simulink library "pmm"  (R2021b)
settings: Solver=VariableStepAuto  StartTime=0.0  StopTime=10.0  RelTol=1e-3
undefined symbols (not defined in the file or in its folder): APMM_CoolgFanActCurr_X_pct, APMM_EWP1Curr_X_c, APMM_EWP3Curr_X_c, APMM_LVBattChktime_X_enum, APMM_LVBattChrgtime_X_enum, APMM_LVChrgLv24V_X_mV, APMM_LVChrgLv_X_mV, ENUM_ANTITHEFT_ALARM, ENUM_ANTITHEFT_ARM, ENUM_ANTITHEFT_DISARM, ENUM_ANTITHEFT_WAIT, ENUM_CHRGPLUGSTA_NONE, ENUM_CRASHSTATE_NOCRASH, ENUM_DCDCFAULTSTA_ANYFAULTLV1, ENUM_DCDCFAULTSTA_ANYFAULTLV2, ENUM_DRIVETRAIN_AWD, ENUM_DRIVETRAIN_FWD, ENUM_DRIVETRAIN_RWD, ENUM_EBSBRKSW_PRESSED, ENUM_GEARACTUALPOSN_D, ENUM_GEARACTUALPOSN_N, ENUM_GEARACTUALPOSN_P, ENUM_GEARACTUALPOSN_R, ENUM_HVBATTREADYPRE_READY, ENUM_PDKEYRAWLULOCK_INLOCK, ENUM_PDKEYRAWLULOCK_INUNLOCK, ENUM_PDKEYRAWPS_INPS, ENUM_PDKEYSTA_LOCK, ENUM_PDKEYSTA_PS, ENUM_PDKEYSTA_UNAVALIABLE, ENUM_PDKEYSTA_UNLOCK, ENUM_POWERSTA_OFF, ENUM_POWERSTA_OFFA, ENUM_POWERSTA_OFFC, ENUM_POWERSTA_ON, ENUM_POWERSTA_READY, ENUM_POWERSTA_STANDBY, ENUM_PWRSTASW_PWRUP, ENUM_PWRSTASW_READY, FALSE, KPMM_AllDoorClosedHoldTime_s, KPMM_APSAllowThd_pct, KPMM_BattDownFailtime_s, KPMM_BattUpFailtime_s, KPMM_BattUpResetRty_cnt, KPMM_BattUpResetSW_flg, KPMM_BattUpResetTO_s, KPMM_BattUpRstDlyTO_s, KPMM_BrakeSWHoldTime_s, KPMM_ChrgPlugHoldTime_s, KPMM_DCDCDisableFailtime_s, KPMM_DCDCEnableFailtime_s, KPMM_DCDCVSET_V, KPMM_DCDCVSETLVChrg_V, KPMM_DoorSWHoldTime_s, KPMM_DriverSafetyChkFailtime_s, KPMM_DrivetrainSelect_enum_ovrdflg, KPMM_DrivetrainSelect_enum_ovrdval, KPMM_FDADC12VDetAccu_s, KPMM_FDADC12VDetAccuIntval_s ... (+60)
libraries: simulink x35, hcu_lib x13
(part 2 of 6)

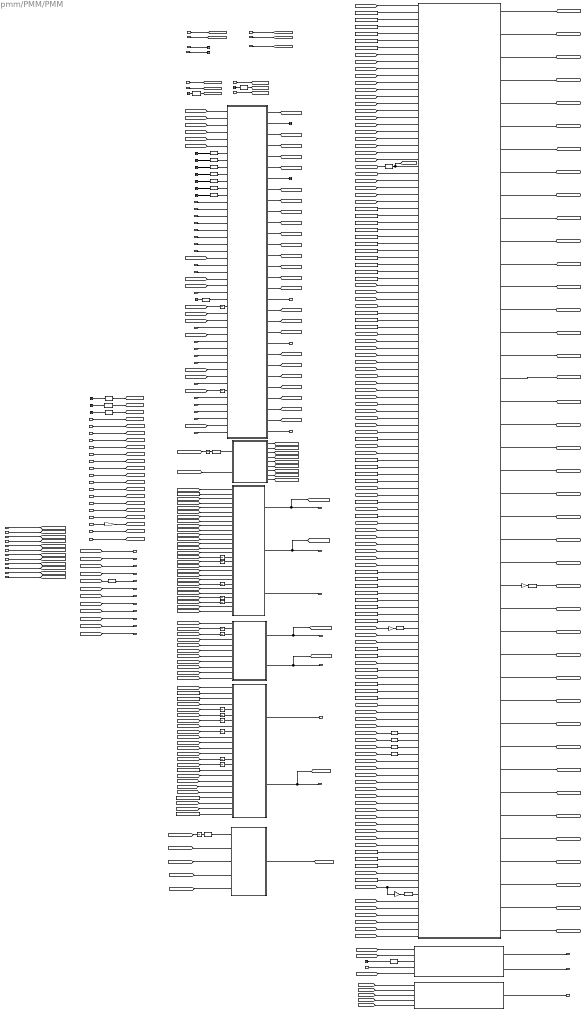
== system pmm/PMM/PMM ==
  note: BMS
  note: PEU
  note: 0 = open; 1 = close
  task_time_s : Inport
  VINP_SeatSW_flg : Inport  Port=2
  VINP_HoodSW_flg : Inport  Port=3
  VINP_TailgateSW_flg : Inport  Port=4
  VINP_PBSWGPIO_flg : Inport  Port=5
  VINP_IVIPwroffreq_flg : Inport  Port=6
  VINP_IVITriggerreq_flg : Inport  Port=7
  VINP_OFFACMODE_enum : Inport  Port=8
  VINP_AVMOFFRecButt_flg : Inport  Port=9
  VINP_SchedChgwake_flg : Inport  Port=10
  VINP_SchedChgbutt_flg : Inport  Port=11
  VINP_PWCONTINUEUSE_flg : Inport  Port=12
  VINP_DCDCReady4Pre_flg : Inport  Port=13
  VINP_DCDCEnabled_flg : Inport  Port=14
  VINP_OBCEnabled_flg : Inport  Port=15
  VINP_OBCReady4Pre_flg : Inport  Port=16
  VINP_OBCFaultStatus_enum : Inport  Port=17
  VINP_DCDCAuxVolt_V : Inport  Port=18
  VINP_RrMCUDCBusVolt_V : Inport  Port=19
  VINP_RrMCUDischrgSta_flg : Inport  Port=20
  VINP_RrMCUEnaSta_flg : Inport  Port=21
  VINP_RrMCUErr_enum : Inport  Port=22
  VINP_RrMCUReady4Pre_flg : Inport  Port=23
  VINP_RrMCUReady_flg : Inport  Port=24
  VINP_RrMCUTemp_C : Inport  Port=25
  VINP_HVBattReady4Pre_enum : Inport  Port=26
  VINP_ChrgPlugSta_enum : Inport  Port=27
  VINP_BMSREADY_flg : Inport  Port=28
  VINP_HVILSta_flg : Inport  Port=29
  VINP_HVBContactorSta_flg : Inport  Port=30
  VINP_ExtChrgSta_enum : Inport  Port=31
  VINP_HVBattSOC_pct : Inport  Port=32
  VINP_RrTMSpd_rpm : Inport  Port=33
  VINP_OBCPluginSta_flg : Inport  Port=34
  VINP_BMSWarn5_flg : Inport  Port=35
  VINP_BMSWarn6_flg : Inport  Port=36
  VINP_BMSWarn7_flg : Inport  Port=37
  VINP_BMSWarn8_flg : Inport  Port=38
  VINP_HVBPreheatPrecoolSta_enum : Inport  Port=39
  VINP_DCDCFaultSta_enum : Inport  Port=40
  VINP_CANMsgValidBMS5_flg : Inport  Port=41
  VINP_CANMsgValidBMS3_flg : Inport  Port=42
  VINP_RrEDURealTMTq_Nm : Inport  Port=43
  VINP_DCDCAuxCur_A : Inport  Port=44
  VINP_V2LSta_enum : Inport  Port=45
  VINP_LVBattDet12V_V : Inport  Port=46
  VINP_PDKeyAreaPS_flg : Inport  Port=47
  VINP_PDKeyAreaLockUnlock_flg : Inport  Port=48
  VINP_CANMsgValidDKC1_flg : Inport  Port=49
  VINP_PowerOffTSet_cnt : Inport  Port=50
  VINP_RePwrReqTbox_enum : Inport  Port=51
  VTQD_GearActualPosn_enum : Inport  Port=52
  VTQD_PBWLockTO_flg : Inport  Port=53
  VBCM_AntitheftSta_enum : Inport  Port=54
  VINP_AllowMovThd_OTA_enum : Inport  Port=55
  VINP_PwrReq_OTA_enum : Inport  Port=56
  VINP_DrivetrainSelect_enum : Inport  Port=57
  VINP_EvccAplusPwrUpReq_flg : Inport  Port=58
  VDHP_ActAPSPosn_pct : Inport  Port=59
  VDHP_EAPS12RangeSta_enum : Inport  Port=60
  VINP_FDEWP1Cmd_enum : Inport  Port=61
  VINP_FDEWP3Cmd_enum : Inport  Port=62
  VINP_CoolgFanActDuty_pct : Inport  Port=63
  VINP_PowerOffTSetDKC_enum : Inport  Port=64
  VINP_RePwrReqDKCT_enum : Inport  Port=65
  VDKC_KeyAreaLockUnlock_enum : Inport  Port=66
  VDKC_KeyAreaPS_enum : Inport  Port=67
  VINP_FASpeed_kph : Inport  Port=68
  VINP_PDUDCDCRlySta_enum : Inport  Port=69
  VINP_PDUEACRlySta_enum : Inport  Port=70
  VINP_PDUEHPSRlySta_enum : Inport  Port=71
  VINP_DCDCEnSta_enum : Inport  Port=72
  VINP_EACEnSta_enum : Inport  Port=73
  VINP_EHPSEnSta_enum : Inport  Port=74
  VINP_EBSBrakeSW_enum : Inport  Port=75
  VINP_PDUSelfChkSta_flg : Inport  Port=76
  VINP_LVBattDet24V_V : Inport  Port=77
  VINP_CANMsgValidDCDCStatus2_flg : Inport  Port=78
  VINP_FDDoorOpen_enum : Inport  Port=79
  VACC_EACPreSelfChkSta_flg : Inport  Port=80
  BoringSpec : Subsystem
  Cast To Boolean : DataTypeConversion  OutDataTypeStr=boolean
  Cast To Boolean1 : DataTypeConversion  OutDataTypeStr=boolean
  Cast To Boolean2 : DataTypeConversion  OutDataTypeStr=boolean
  Constant : Constant  Value=KPMM_LVBattChkOKStdT_s
  Constant1 : Constant  Value=KPMM_LVBattThd_V
  Constant10 : Constant  Value=KPMM_OBCDisableFailtime_s
  Constant11 : Constant  Value=KPMM_DriverSafetyChkFailtime_s
  Constant12 : Constant  Value=KPMM_FDADC12VDetAccu_s
  Constant13 : Constant  Value=KPMM_PrechrgChkFailtime_s
  Constant14 : Constant  Value=KPMM_FirstLVCheckHoldT_s
  Constant15 : Constant  Value=KPMM_MLvSafetyFailtime_s
  Constant16 : Constant  Value=KPMM_MCUDisChrgFailtime_s
  Constant17 : Constant  Value=KPMM_DCDCVSET_V
  Constant18 : Constant  Value=KPMM_OFFStaByPassLVBatt_flg
  Constant19 : Constant  Value=KPMM_SilentChrgReq_flg_ovrdflg
  Constant2 : Constant  Value=KPMM_PwrStaStdTO_s
  Constant20 : Constant  Value=KPMM_DCDCEnableFailtime_s
  Constant21 : Constant  Value=KPMM_BattDownFailtime_s
  Constant22 : Constant  Value=KPMM_MCUDisableFailtime_s
  Constant23 : Constant  Value=KPMM_APSAllowThd_pct
  Constant24 : Constant  Value=KPMM_DCDCDisableFailtime_s
  Constant25 : Constant  Value=KPMM_SilentChrgReq_flg_ovrdval
  Constant26 : Constant  Value=KPMM_HVBattSOCThd_pct
  Constant27 : Constant  Value=KPMM_HVSOCWarnThd_pct
  Constant28 : Constant  Value=KPMM_HVBattSOCPwrDwnThd_pct
  Constant29 : Constant  Value=KPMM_HVSOCWarnThd_pct
  Constant3 : Constant  Value=KPMM_HVBattSOCThd_pct
  Constant30 : Constant  Value=KPMM_OffA2OffTime_s
  Constant31 : Constant  Value=KPMM_PluginVehSpdThd_kph
  Constant32 : Constant  Value=KPMM_LVChrgCurrMthd_flg
  Constant33 : Constant  Value=KPMM_LVChrgHoldT_s
  Constant34 : Constant  Value=KPMM_SysBaseCurr_A
  Constant35 : Constant  Value=KPMM_HVSOCWarnTime_s
  Constant36 : Constant  Value=KPMM_SilentChrgReqTO_s
  Constant37 : Constant  Value=KPMM_PwrStaONTOPop_s
  Constant38 : Constant  Value=KPMM_LVBattChkWakehold_s
  Constant39 : Constant  Value=KPMM_LVBattOFFSlpThd_mV
  Constant4 : Constant  Value=KPMM_HVBSOCOffStaChkFailtime_s
  Constant40 : Constant  Value=KPMM_OFFLVBattChkRetry_cnt
  Constant41 : Constant  Value=KPMM_SysPwrDownDbns_s
  Constant42 : Constant  Value=KPMM_BattUpResetRty_cnt
  Constant43 : Constant  Value=KPMM_BattUpResetSW_flg
  Constant44 : Constant  Value=KPMM_BattUpResetTO_s
  Constant45 : Constant  Value=KPMM_BattUpRstDlyTO_s
  Constant46 : Constant  Value=KPMM_HoodOffChkFailtime_s
  Constant47 : Constant  Value=KPMM_FDADC24VDetAccu_s
  Constant48 : Constant  Value=KPMM_FDADC24VDetAccuIntval_s
  Constant49 : Constant  Value=KPMM_LVBattOFFSlpThd24V_mV
  Constant5 : Constant  Value=KPMM_HVBSOCOFFCStaChkFailtime_s
  Constant50 : Constant  Value=KPMM_LVBattThd24V_V
  Constant6 : Constant  Value=KPMM_FDADC12VDetAccuIntval_s
  Constant7 : Constant  Value=KPMM_OBCPreChgChkFailtime_s
  Constant8 : Constant  Value=KPMM_SafetyChkFailtime_s
  Constant9 : Constant  Value=KPMM_BattUpFailtime_s  OutDataTypeStr=single
  DCDC output volt setpoint judgment : Subsystem
  Data Type Conversion : DataTypeConversion
  Data Type Conversion1 : DataTypeConversion
  Data Type Conversion{3,5,10,15} (4 alike) : DataTypeConversion  OutDataTypeStr=uint8
  Data Type Conversion{7..9,11..12} (5 alike) : DataTypeConversion  OutDataTypeStr=boolean
  Data Type Conversion{2,4,6,13..14,16} (6 alike) : DataTypeConversion  OutDataTypeStr=single
  Data Type Conversion39 : DataTypeConversion
  Detect Decrease : simulink/Logic and Bit Operations/Detect Decrease  vinit=0.0  OutDataTypeStr=boolean
  Detect Increase : simulink/Logic and Bit Operations/Detect Increase  vinit=0.0  OutDataTypeStr=boolean
  Detect Increase1 : simulink/Logic and Bit Operations/Detect Increase  vinit=0.0  OutDataTypeStr=boolean
  Detect Increase2 : simulink/Logic and Bit Operations/Detect Increase  vinit=0.0  OutDataTypeStr=boolean
  Gain : Gain  Gain=MIN2SEC
  Gain1 : Gain  Gain=1000
  Gain2 : Gain  Gain=0.001
  Gain3 : Gain  Gain=1000
  Ground{,1..13} (14 alike) : Ground
  MCU_EnaReq_Control : Subsystem
  PMMDataConvert : Subsystem  AncestorBlock=pmm/PMM/PowerModeManagement/PMMDataConvert
  PMM_State_Machine : Stateflow chart  TreatAsAtomicUnit=on
      settings: PortSchema="{\"entries\":[{\"content\":{\"sides\":[{\"content\":{\"connectorIds\":[\"In1\",\"In2\",\"In3\",\"In4\",\"In5\",\"In6\",\"In7\",\"In8\",\"In9\",\"In10\",\"In11\",\"In12\",\"In13\",\"In14\",\"In15\",\"In16\",\"In17\",\"In18\",\"In19\",\"In20\",\"In21\",\"In22\",\"In23\",\"In24\",\"In25\",\"In26\",\"In27\",\"In28\",\"In29\",\"In30\",\"In31\",\"In32\",\"In33\",\"In34\",\"In35\",\"In36\",\"In37\",\"In38\",\"In39\",\"In40\",\"In41\",\"In42\",\"In43\",\"In44\",\"In45\",\"In46\",\"In47\",\"In48\",\"In49\",\"In50\",\"In52\",\"In53\",\"In54\",\"In55\",\"In56\",\"In57\",\"In58\",\"In51\",\"In59\",\"In60\",\"In61\",\"In62\",\"In63\",\"In65\",\"In66\",\"In67\",\"In68\",\"In69\",\"In70\",\"In73\",\"In74\",\"In71\",\"In72\",\"In64\",\"In75\",\"In76\",\"In77\",\"In78\",\"In79\",\"In80\",\"In81\",\"In82\",\"In83\",\"In84\",\"In85\",\"In86\",\"In87\",\"In88\",\"In89\",\"In90\",\"In96\",\"In97\",\"In98\",\"In99\",\"In100\",\"In95\",\"In91\",\"In92\",\"In93\",\"In94\",\"In101\",\"In102\",\"In103\",\"In104\",\"In105\",\"In106\",\"In107\",\"In108\",\"In109\",\"In110\",\"In111\",\"In112\",\"In113\",\"In114\",\"In115\",\"In116\",\"In117\",\"In118\",\"In119\",\"In120\",\"In121\",\"In123\",\"In124\",\"In125\",\"In126\",\"In127\",\"In128\",\"In122\",\"In129\",\"In130\",\"In131\",\"In132\",\"In133\",\"In134\"]},\"type\":\"ConnectorPlacement.EquallySpacedRectSide\",\"uuid\":\"8ab1b0ff-73ed-4b41-8f3f-fcf16c31188d\"},{\"content\":{\"connectorIds\":[\"Out1\",\"Out2\",\"Out3\",\"Out4\",\"Out5\",\"Out6\",\"Out7\",\"Out8\",\"Out9\",\"Out10\",\"Out11\",\"Out12\",\"Out13\",\"Out14\",\"Out17\",\"Out18\",\"Out19\",\"Out20\",\"Out21\",\"Out22\",\"Out23\",\"Out24\",\"Out25\",\"Out26\",\"Out27\",\"Out28\",\"Out29\",\"Out30\",\"Out31\",\"Out32\",\"Out33\",\"Out34\",\"Out35\",\"Out15\",\"Out16\",\"Out36\",\"Out37\",\"Out38\",\"Out40\",\"Out41\",\"Out39\"],\"side\":\"RIGHT\"},\"type\":\"ConnectorPlacement.EquallySpacedRectSide\",\"uuid\":\"e75ad163-33ee-46d6-b33a-670f57cb3f5e\"},{\"content\":{\"connectorIds\":[],\"side\":\"TOP\"},\"type\":\"ConnectorPlacement.EquallySpacedRectSide\",\"uuid\":\"84c68278-d5af-48d1-859e-0f05090acbaa\"}]},\"type\":\"ConnectorPlacement.EquallySpacedConnector\",\"uuid\":\"278d3476-0e07-485b-a357-39a0667eafe4\"}],\"packageUris\":[\"http://schema.mathworks.com/mf0/Connector/R2020b\"],\"version\":\"1.0\"}"
  PushButton_Handle : Subsystem
  RequirementManagementForPowerDown : Stateflow chart  TreatAsAtomicUnit=on
  RequirementManagementForPowerStateConstrain : Stateflow chart  TreatAsAtomicUnit=on
      settings: PortSchema="{\"entries\":[{\"content\":{\"sides\":[{\"content\":{\"connectorIds\":[\"In1\",\"In2\",\"In11\",\"In3\",\"In4\",\"In5\",\"In6\",\"In7\",\"In8\",\"In9\",\"In10\"]},\"type\":\"ConnectorPlacement.EquallySpacedRectSide\",\"uuid\":\"c4039c9e-34d9-4d76-8a20-7739646b6da6\"},{\"content\":{\"connectorIds\":[\"Out1\",\"Out2\"],\"side\":\"RIGHT\"},\"type\":\"ConnectorPlacement.EquallySpacedRectSide\",\"uuid\":\"63e3e661-9024-478e-a9c0-8e66b2c0118c\"},{\"content\":{\"connectorIds\":[],\"side\":\"TOP\"},\"type\":\"ConnectorPlacement.EquallySpacedRectSide\",\"uuid\":\"6c94eba6-19b8-417a-9a11-c61323531ba8\"}]},\"type\":\"ConnectorPlacement.EquallySpacedConnector\",\"uuid\":\"e4d90d6b-0647-4724-8d20-4a3edeab4c97\"}],\"packageUris\":[\"http://schema.mathworks.com/mf0/Connector/R2020b\"],\"version\":\"1.0\"}"
  RequirementManagementForPowerUp : Stateflow chart  TreatAsAtomicUnit=on
  Terminator{,1..3} (4 alike) : Terminator
  Unit Delay{,1..16} (17 alike) : UnitDelay  SampleTime=-1  HasFrameUpgradeWarning=on
  VPMM_PowerUpState_enum : Outport
  VPMM_PowerDownState_enum : Outport  Port=2
  VPMM_PowerUpFault_enum : Outport  Port=3
  VPMM_PowerDownFault_enum : Outport  Port=4
  VPMM_ActiveDischargeReq_flg : Outport  Port=5
  VPMM_DCDCEnaReq_flg : Outport  Port=6
  VPMM_DCDCVoltSetpoint_V : Outport  Port=7
  VPMM_HVBatCnctReq_flg : Outport  Port=8
  VPMM_HVSysReadyToCharge_enum : Outport  Port=9
  VPMM_PowerSta_enum : Outport  Port=10
  VPMM_LVPwrSta_flg : Outport  Port=11
  VPMM_HVPwrSta_flg : Outport  Port=12
  VPMM_SysPowerMode_enum : Outport  Port=13
  VPMM_FrMCUEnaReq_flg : Outport  Port=14
  VPMM_RrMCUEnaReq_flg : Outport  Port=15
  VPMM_DrivetrainSelect_enum : Outport  Port=16
  VPMM_DrSeatSta_enum : Outport  Port=17
  VPMM_PwrStaSelect_enum : Outport  Port=18
  VPMM_PwrStaConstraint_enum : Outport  Port=19
  VPMM_TCountSta_enum : Outport  Port=20
  VPMM_PwrUpReq_enum : Outport  Port=21
  VPMM_PwrDownReq_enum : Outport  Port=22
  VPMM_LowSOCWarn_enum : Outport  Port=23
  VPMM_ReVehThdChkSta_enum : Outport  Port=24
  VPMM_LVSysErrPwrOutErr_flg : Outport  Port=25
  VPMM_EvccAplusPwrUpReq_flg : Outport  Port=26
  VPMM_PwrStaONTOPopReq_flg : Outport  Port=27
  VPMM_IVIPwrStaONTOPopT_s : Outport  Port=28
  VPMM_LVChrgHoldTtimer_s : Outport  Port=29
  VPMM_LVBattChrgTimeCnt_s : Outport  Port=30
  VPMM_SilentChkAllowSleep_flg : Outport  Port=31
  VPMM_TimerAllowSleep_flg : Outport  Port=32
  VPMM_FDADC12VDetAvg_mV : Outport  Port=33
  VPMM_PMMAllowECUSleep_flg : Outport  Port=34
  VPMM_LVSilentChrgSta_enum : Outport  Port=35
  VPMM_LVSilentChrgReq_flg : Outport  Port=36
  VPMM_LVSilentChrgLv_enum : Outport  Port=37
  VPMM_LVBattChktime_s : Outport  Port=38
  VPMM_SafetyChkMLv_flg : Outport  Port=39
  VPMM_SafetyChkHLv_flg : Outport  Port=40
  VPMM_HVChrgPreActionErrSta_enum : Outport  Port=41
  VPMM_MCUReady_flg : Outport  Port=42
  VPMM_MCUReady4Pre_flg : Outport  Port=43
  VPMM_CtrlFrPwrStbA1P_flg : Outport  Port=44
  VPMM_CtrlFrRC1_flg : Outport  Port=45
  VPMM_CtrlFrBMSCCUCIR_flg : Outport  Port=46
  VPMM_CtrlFrEDUINVERTER_flg : Outport  Port=47
  VPMM_HWResetSta_enum : Outport  Port=48
  VPMM_CtrlDrPwrStbA2_flg : Outport  Port=49
  VPMM_PwrStaTOSta_enum : Outport  Port=50
  VPMM_PMMAllowNMSleep_flg : Outport  Port=51
  VPMM_DCDCRlyDem_enum : Outport  Port=52
  VPMM_EACRlyDem_enum : Outport  Port=53
  VPMM_EHPSRlyDem_enum : Outport  Port=54
  VPMM_DCDCEnDem_enum : Outport  Port=55
  wires:
  PMM_State_Machine/16(VPMM_PwrStaTOSta_enum) -> [VPMM_PwrStaTOSta_enum]  "VPMM_PwrStaTOSta_enum"
  PMM_State_Machine/17(VPMM_Sched_ChgTOSta_enum) -> [VPMM_Sched_ChgTOSta_enum]  "VPMM_Sched_ChgTOSta_enum"
  PMM_State_Machine/15(VPMM_LVSilentChrgReq_flg) -> [VPMM_LVSilentChrgReq_flg]  "VPMM_LVSilentChrgReq_flg"
  PMM_State_Machine/18(VPMM_LVSilentChrgReqStd_flg) -> [VPMM_LVSilentChrgReqStd_flg]  "VPMM_LVSilentChrgReqStd_flg"
  VDHP_EAPS12RangeSta_enum/1 -> PMM_State_Machine/65(VDHP_EAPS12RangeSta_enum)
  Constant2/1 -> PMM_State_Machine/64(KPMM_PwrStaStdTO_s)
  Constant/1 -> PMM_State_Machine/63(KPMM_LVBattChkOKStdT_s)
  [VINP_EvccAplusPwrUpReq_flg] -> RequirementManagementForPowerUp/24(VINP_EvccAplusPwrUpReq_flg)
  VINP_EvccAplusPwrUpReq_flg/1 -> [VINP_EvccAplusPwrUpReq_flg]
  [VPMM_LVSilentChrgReqStd_flg] -> Unit Delay8/1
  Unit Delay8/1 -> RequirementManagementForPowerUp/25(VPMM_LVSilentChrgReqStd_flg)
  [VINP_ChrgPlugSta_enum] -> RequirementManagementForPowerUp/23(VINP_ChrgPlugSta_enum)
  [VINP_PwrReq_OTA_enum] -> PMM_State_Machine/61(VINP_PwrReq_OTA_enum)
  Unit Delay7/1 -> RequirementManagementForPowerDown/14(VPMM_Sched_ChgTOSta_enum)
  [VPMM_Sched_ChgTOSta_enum] -> Unit Delay7/1
  [VPMM_PowerUpState_enum] -> Unit Delay1/1
  Unit Delay1/1 -> RequirementManagementForPowerUp/22(VPMM_PowerUpState_enum)
  [task_time_s] -> RequirementManagementForPowerUp/1(task_time_s)
  [VPMM_DrivetrainSelect_enum] -> MCU_EnaReq_Control/5(VPMM_DrivetrainSelect_enum)
  MCU_EnaReq_Control/2(VPMM_RrMCUEnaReq_flg) -> VPMM_RrMCUEnaReq_flg/1  "VPMM_RrMCUEnaReq_flg"
  MCU_EnaReq_Control/1(VPMM_FrMCUEnaReq_flg) -> VPMM_FrMCUEnaReq_flg/1  "VPMM_FrMCUEnaReq_flg"
  Unit Delay6/1 -> PMMDataConvert/29(VPMM_PowerSta_enum)
  Unit Delay5/1 -> RequirementManagementForPowerDown/5(VPMM_PowerSta_enum)
  Unit Delay4/1 -> RequirementManagementForPowerStateConstrain/2(VPMM_PowerSta_enum)
  Unit Delay3/1 -> RequirementManagementForPowerUp/16(VPMM_LVSilentChrgReq_flg)
  [VPMM_AllDoorClosed_flg] -> RequirementManagementForPowerUp/9(VPMM_AllDoorClosed_flg)
  Unit Delay2/1 -> RequirementManagementForPowerDown/7(VPMM_PwrStaTOSta_enum)
  Unit Delay/1 -> RequirementManagementForPowerUp/17(VPMM_PowerSta_enum)
  VINP_CANMsgValidBMS3_flg/1 -> PMM_State_Machine/60(VINP_CANMsgValidBMS3_flg)
  PMM_State_Machine/14(VPMM_LVBattChktime_s) -> VPMM_LVBattChktime_s/1  "VPMM_LVBattChktime_s"
  [VPMM_PwrUpReq_enum] -> PMM_State_Machine/59(VPMM_PwrUpReq_enum)
  [VPMM_PwrStaSelect_enum] -> PMM_State_Machine/58(VPMM_PwrStaSelect_enum)
  [VPMM_PwrStaConstraint_enum] -> PMM_State_Machine/57(VPMM_PwrStaConstraint_enum)
  [VPMM_PwrDownReq_enum] -> PMM_State_Machine/56(VPMM_PwrDownReq_enum)
  VINP_AllowMovThd_OTA_enum/1 -> PMM_State_Machine/55(VINP_AllowMovThd_OTA_enum)
  [VINP_PwrReq_OTA_enum] -> RequirementManagementForPowerDown/11(VINP_PwrReq_OTA_enum)
  [VINP_PowerOffTSetDKC_enum] -> RequirementManagementForPowerDown/10(VINP_PowerOffTSetDKC_enum)
  [VINP_RePwrReqDKCT_enum] -> RequirementManagementForPowerDown/13(VINP_RePwrReqDKCT_enum)
  [VINP_RePwrReqTbox_enum] -> RequirementManagementForPowerDown/12(VINP_RePwrReqTbox_enum)
  [VPMM_TCountSta_enum] -> Unit Delay12/1
  [VPMM_PowerOffTSet_s] -> RequirementManagementForPowerDown/8(VPMM_PowerOffTSet_s)
  [VPMM_PwrStaTOSta_enum] -> Unit Delay2/1
  [VINP_HVBattSOC_pct] -> RequirementManagementForPowerDown/4(VINP_HVBattSOC_pct)
  [VINP_RePwrReqTbox_enum] -> RequirementManagementForPowerUp/21(VINP_RePwrReqTbox_enum)
  [VINP_RePwrReqDKCT_enum] -> RequirementManagementForPowerUp/20(VINP_RePwrReqDKCT_enum)
  VINP_PowerOffTSetDKC_enum/1 -> [VINP_PowerOffTSetDKC_enum]
  VINP_RePwrReqDKCT_enum/1 -> [VINP_RePwrReqDKCT_enum]
  VINP_RePwrReqTbox_enum/1 -> [VINP_RePwrReqTbox_enum]
  [VINP_PwrReq_OTA_enum] -> RequirementManagementForPowerUp/19(VINP_PwrReq_OTA_enum)
  VINP_PwrReq_OTA_enum/1 -> [VINP_PwrReq_OTA_enum]
  [VTQD_GearActualPosn_enum] -> RequirementManagementForPowerUp/18(VTQD_GearActualPosn_enum)
  [VTQD_GearActualPosn_enum] -> PMM_State_Machine/29(VTQD_GearActualPosn_enum)
  VTQD_GearActualPosn_enum/1 -> [VTQD_GearActualPosn_enum]
  [VPMM_DetectDoorOpened_flg] -> RequirementManagementForPowerUp/15(VPMM_DetectDoorOpened_flg)
  [VPMM_ChrgPlugInRisingEdge_flg] -> RequirementManagementForPowerUp/14(VPMM_ChrgPlugInRisingEdge_flg)
  [VPMM_LVSilentChrgReq_flg] -> Unit Delay3/1
  [VPMM_BrkPedalRisingEdge_flg] -> RequirementManagementForPowerUp/13(VPMM_BrkPedalRisingEdge_flg)
  [VBCM_AntitheftSta_enum] -> RequirementManagementForPowerUp/10(VBCM_AntitheftSta_enum)
  [VINP_HVBattSOC_pct] -> RequirementManagementForPowerUp/4(VINP_HVBattSOC_pct)
  [VINP_HVBattSOC_pct] -> PMM_State_Machine/28(VINP_HVBattSOC_pct)
  VINP_HVBattSOC_pct/1 -> [VINP_HVBattSOC_pct]
  VINP_SchedChgbutt_flg/1 -> PMM_State_Machine/51(VINP_SchedChgbutt_flg)
  [VINP_TailgateSW_flg] -> RequirementManagementForPowerUp/6(VINP_TailgateSW_flg)
  [VINP_HoodSW_flg] -> RequirementManagementForPowerUp/5(VINP_HoodSW_flg)
  [VINP_HoodSW_flg] -> PMM_State_Machine/54(VINP_HoodSW_flg)
  VINP_TailgateSW_flg/1 -> [VINP_TailgateSW_flg]
  VINP_HoodSW_flg/1 -> [VINP_HoodSW_flg]
  [VINP_HVBPreheatPrecoolSta_enum] -> RequirementManagementForPowerUp/3(VINP_HVBPreheatPrecoolSta_enum)
  VINP_HVBPreheatPrecoolSta_enum/1 -> [VINP_HVBPreheatPrecoolSta_enum]
  [VPMM_PwrStaConstraint_enum] -> Unit Delay11/1
  [VPMM_BrkPedalPressed_flg] -> RequirementManagementForPowerUp/12(VPMM_BrkPedalPressed_flg)
  [VPMM_BMSWarm_flg] -> RequirementManagementForPowerUp/11(VPMM_BMSWarn_flg)
  [VPMM_PowerSta_enum] -> Unit Delay/1
  [VPMM_PowerSta_enum] -> Unit Delay5/1
  [VPMM_PowerSta_enum] -> Unit Delay4/1
  [task_time_s] -> RequirementManagementForPowerDown/1(task_time_s)
  [task_time_s] -> RequirementManagementForPowerStateConstrain/1(task_time_s)
  Constant30/1 -> RequirementManagementForPowerDown/3(KPMM_OffA2OffTime_s)
  Constant29/1 -> RequirementManagementForPowerDown/2(KPMM_HVSOCWarnThd_pct)
  Constant26/1 -> RequirementManagementForPowerUp/2(KPMM_HVBattSOCThd_pct)
  [VBCM_AntitheftSta_enum] -> PMMDataConvert/2(VBCM_AntitheftSta_enum)
  VBCM_AntitheftSta_enum/1 -> [VBCM_AntitheftSta_enum]
  [VPMM_MCUDCBusMaxVolt_V] -> PMM_State_Machine/52(VPMM_MCUDCBusMaxVolt_V)
  [VINP_DrDoorSW_flg] -> PMM_State_Machine/53(VINP_DrDoorSW_flg)
  [VPMM_SeatSWRisingEdge_flg] -> PMM_State_Machine/50(VPMM_SeatSWRisingEdge_flg)
  [VPMM_ChrgPlugOutFallingEdge_flg] -> PMM_State_Machine/49(VPMM_ChrgPlugFallingEdge_flg)
  VINP_OBCPluginSta_flg/1 -> PMM_State_Machine/48(VINP_OBCPluginSta_flg)
  Constant18/1 -> PMM_State_Machine/47(KPMM_OFFStaByPassLVBatt_flg)
  Constant25/1 -> PMM_State_Machine/46(KPMM_SilentChrgReq_flg_ovrdval)
  Constant19/1 -> PMM_State_Machine/45(KPMM_SilentChrgReq_flg_ovrdflg)
  VTQD_PBWLockTO_flg/1 -> PMM_State_Machine/44(VTQD_EnterPGearFail_flg)
  [VPMM_AllDoorCloseRisingEdge_flg] -> PMM_State_Machine/43(VPMM_AllDoorCloseRisingEdge_flg)
  [VINP_DCDCEnabled_flg] -> PMM_State_Machine/41(VINP_DCDCEnabled_flg)
  Constant17/1 -> PMM_State_Machine/40(KPMM_DCDCVSET_V)
  Constant16/1 -> PMM_State_Machine/39(KPMM_MCUDisChrgFailtime_s)
  Constant15/1 -> PMM_State_Machine/38(KPMM_MLvSafetyFailtime_s)
  [VPMM_PDKeySta_enum] -> PMM_State_Machine/26(VPMM_PDKeySta_enum)
  Constant13/1 -> PMM_State_Machine/37(KPMM_PrechrgChkFailtime_s)
  [VINP_SeatSW_flg] -> PMM_State_Machine/27(VINP_SeatSW_flg)
  Constant11/1 -> PMM_State_Machine/36(KPMM_DriverSafetyChkFailtime_s)
  Constant8/1 -> PMM_State_Machine/35(KPMM_SafetyChkFailtime_s)
  Constant7/1 -> PMM_State_Machine/34(KPMM_OBCPreChgChkFailtime_s)
  Constant1/1 -> PMM_State_Machine/30(KPMM_LVBattThd_V)
  Constant5/1 -> PMM_State_Machine/33(KPMM_HVBSOCOFFCStaChkFailtime_s)
  Constant3/1 -> PMM_State_Machine/31(KPMM_HVBattSOCThd_pct)
  Constant4/1 -> PMM_State_Machine/32(KPMM_HVBSOCOffStaChkFailtime_s)
  VINP_IVITriggerreq_flg/1 -> PMM_State_Machine/25(VINP_IVITriggerreq_flg)
  [VPMM_SafetyChkMLv_flg] -> PMM_State_Machine/23(VPMM_SafetyChkMLv_flg)
  [VPMM_SafetyChkHLv_flg] -> PMM_State_Machine/22(VPMM_SafetyChkHLv_flg)
  [VINP_OBCEnabled_flg] -> PMM_State_Machine/21(VINP_OBCEnabled_flg)
  [VINP_OBCReady4Pre_flg] -> PMM_State_Machine/20(VINP_OBCReady4Pre_flg)
  [VPMM_BrkPedalRisingEdge_flg] -> PMM_State_Machine/19(VPMM_BrkPedalRisingEdge_flg)
  [VPMM_MCUReady_flg] -> PMM_State_Machine/18(VPMM_MCUReady_flg)
  [VPMM_BrkPedalPressed_flg] -> PMM_State_Machine/17(VPMM_BrkPedalPressed_flg)
  [VPMM_AllDoorClosed_flg] -> PMM_State_Machine/16(VPMM_AllDoorClosed_flg)
  [VPMM_PreChrgChk_flg] -> PMM_State_Machine/15(VPMM_PreChrgChk_flg)
  [VPMM_MCUEnable_flg] -> PMM_State_Machine/14(VPMM_MCUEnable_flg)
  [VPMM_DetectDoorOpened_flg] -> PMM_State_Machine/13(VPMM_DetectDoorOpened_flg)
  [VINP_HVBContactorSta_flg] -> PMM_State_Machine/12(VINP_HVBContactorSta_flg)
  [VINP_ChrgPlugSta_enum] -> PMM_State_Machine/11(VINP_ChrgPlugSta_enum)
  [VINP_ExtChrgSta_enum] -> PMM_State_Machine/9(VINP_ExtChrgSta_enum)
  [VINP_BMSREADY_flg] -> PMM_State_Machine/8(VINP_BMSREADY_flg)
  Constant10/1 -> PMM_State_Machine/7(KPMM_OBCDisableFailtime_s)
  Constant24/1 -> PMM_State_Machine/6(KPMM_DCDCDisableFailtime_s)
  Constant22/1 -> PMM_State_Machine/5(KPMM_MCUDisableFailtime_s)
  Constant21/1 -> PMM_State_Machine/4(KPMM_BattDownFailtime_s)
  Constant20/1 -> PMM_State_Machine/3(KPMM_DCDCEnableFailtime_s)
  Constant9/1 -> PMM_State_Machine/2(KPMM_BattUpFailtime_s)
  [task_time_s] -> PMM_State_Machine/1(task_time_s)
  RequirementManagementForPowerUp/3(VPMM_ReVehThdChkSta_enum) -> VPMM_ReVehThdChkSta_enum/1  "VPMM_ReVehThdChkSta_enum"
  RequirementManagementForPowerDown/1(VPMM_LowSOCWarn_enum) -> VPMM_LowSOCWarn_enum/1  "VPMM_LowSOCWarn_enum"
  RequirementManagementForPowerDown/2(VPMM_PwrDownReq_enum) -> [VPMM_PwrDownReq_enum], VPMM_PwrDownReq_enum/1  "VPMM_PwrDownReq_enum"
  RequirementManagementForPowerUp/2(VPMM_PwrUpReq_enum) -> [VPMM_PwrUpReq_enum], VPMM_PwrUpReq_enum/1  "VPMM_PwrUpReq_enum"
  RequirementManagementForPowerStateConstrain/2(VPMM_TCountSta_enum) -> VPMM_TCountSta_enum/1, [VPMM_TCountSta_enum]  "VPMM_TCountSta_enum"
  RequirementManagementForPowerStateConstrain/1(VPMM_PwrStaConstraint_enum) -> VPMM_PwrStaConstraint_enum/1, [VPMM_PwrStaConstraint_enum]  "VPMM_PwrStaConstraint_enum"
  RequirementManagementForPowerUp/1(VPMM_PwrStaSelect_enum) -> [VPMM_PwrStaSelect_enum], VPMM_PwrStaSelect_enum/1  "VPMM_PwrStaSelect_enum"
  PMMDataConvert/18(VPMM_DrSeatSta_enum) -> VPMM_DrSeatSta_enum/1
  [VINP_DrDoorSW_flg] -> PMMDataConvert/3(VINP_DrDoorSW_flg)
  Ground9/1 -> Data Type Conversion7/1
  PMMDataConvert/20(VPMM_MCUDCBusMaxVolt_V) -> [VPMM_MCUDCBusMaxVolt_V]
  VINP_RrMCUErr_enum/1 -> PMMDataConvert/17(VINP_RrMCUErr_enum)
  VINP_RrMCUEnaSta_flg/1 -> PMMDataConvert/16(VINP_RrMCUEnaSta_flg)
  VINP_RrMCUDischrgSta_flg/1 -> PMMDataConvert/15(VINP_RrMCUDischrgSta_flg)
  VINP_RrMCUDCBusVolt_V/1 -> PMMDataConvert/14(VINP_RrMCUDCBusVolt_V)
  Ground6/1 -> Data Type Conversion13/1
  Ground5/1 -> Data Type Conversion12/1
  Ground4/1 -> Data Type Conversion11/1
  Ground3/1 -> Data Type Conversion10/1
  Ground2/1 -> Data Type Conversion9/1
  Ground1/1 -> Data Type Conversion8/1
  Ground/1 -> Data Type Conversion14/1
  PMMDataConvert/19(VPMM_BMSWarm_flg) -> [VPMM_BMSWarm_flg]
  VINP_BMSWarn8_flg/1 -> PMMDataConvert/35(VINP_BMSWarn8_flg)
  VINP_BMSWarn7_flg/1 -> PMMDataConvert/34(VINP_BMSWarn7_flg)
  VINP_BMSWarn5_flg/1 -> PMMDataConvert/32(VINP_BMSWarn5_flg)
  [VINP_FrTMSpd_rpm] -> PMMDataConvert/31(VINP_FrTMSpd_rpm)
  [VINP_RrTMSpd_rpm] -> PMMDataConvert/30(VINP_RrTMSpd_rpm)
  Ground7/1 -> Data Type Conversion6/1
  VINP_RrTMSpd_rpm/1 -> [VINP_RrTMSpd_rpm]
  PMMDataConvert/15(VPMM_SeatSWRisingEdge_flg) -> [VPMM_SeatSWRisingEdge_flg]
  PMMDataConvert/14(VPMM_ChrgPlugOutFallingEdge_flg) -> [VPMM_ChrgPlugOutFallingEdge_flg]
  PMMDataConvert/17(VPMM_SafetyChkHLv_flg) -> [VPMM_SafetyChkHLv_flg]
  PMMDataConvert/16(VPMM_SafetyChkMLv_flg) -> [VPMM_SafetyChkMLv_flg]
  PMMDataConvert/13(VPMM_ChrgPlugInRisingEdge_flg) -> [VPMM_ChrgPlugInRisingEdge_flg]
  [VINP_SeatSW_flg] -> PMMDataConvert/26(VINP_SeatSW_flg)
  VINP_SeatSW_flg/1 -> [VINP_SeatSW_flg]
  [VPMM_PowerSta_enum] -> Unit Delay6/1
  Ground13/1 -> Data Type Conversion15/1
  VINP_HVILSta_flg/1 -> PMMDataConvert/27(VINP_HVILSta_flg)
  VINP_OBCFaultStatus_enum/1 -> Terminator/1
  [VPMM_DrivetrainSelect_enum] -> VPMM_DrivetrainSelect_enum/1  "VPMM_DrivetrainSelect_enum"
  PMMDataConvert/12(VPMM_DrivetrainSelect_enum) -> [VPMM_DrivetrainSelect_enum]
  PMMDataConvert/11(VPMM_AllDoorCloseRisingEdge_flg) -> [VPMM_AllDoorCloseRisingEdge_flg]
  VINP_HVBContactorSta_flg/1 -> [VINP_HVBContactorSta_flg]
  VINP_ExtChrgSta_enum/1 -> [VINP_ExtChrgSta_enum]
  VINP_DCDCAuxVolt_V/1 -> Terminator3/1
  task_time_s/1 -> [task_time_s]
  VINP_ChrgPlugSta_enum/1 -> [VINP_ChrgPlugSta_enum]
  VINP_OBCEnabled_flg/1 -> [VINP_OBCEnabled_flg]
  VINP_BMSREADY_flg/1 -> [VINP_BMSREADY_flg]
  VINP_DCDCEnabled_flg/1 -> [VINP_DCDCEnabled_flg]
  VINP_OBCReady4Pre_flg/1 -> [VINP_OBCReady4Pre_flg]
  VINP_HVBattReady4Pre_enum/1 -> PMMDataConvert/23(VINP_HVBattReady4Pre_enum)
  VINP_DCDCReady4Pre_flg/1 -> PMMDataConvert/21(VINP_DCDCReady4Pre_flg)
  VINP_RrMCUTemp_C/1 -> PMMDataConvert/20(VINP_RrMCUTemp_C)
  VINP_RrMCUReady_flg/1 -> PMMDataConvert/19(VINP_RrMCUReady_flg)
  PMM_State_Machine/12(VPMM_HVPwrSta_flg) -> [VPMM_HVPwrSta_flg]  "VPMM_HVPwrSta_flg"
  PMM_State_Machine/11(VPMM_LVPwrSta_flg) -> VPMM_LVPwrSta_flg/1  "VPMM_LVPwrSta_flg"
  PMM_State_Machine/8(VPMM_HVBatCnctReq_flg) -> VPMM_HVBatCnctReq_flg/1  "VPMM_HVBatCnctReq_flg"
  VINP_RrMCUReady4Pre_flg/1 -> PMMDataConvert/18(VINP_RrMCUReady4Pre_flg)
  PMM_State_Machine/6(VPMM_DCDCEnaReq_flg) -> VPMM_DCDCEnaReq_flg/1  "VPMM_DCDCEnaReq_flg"
  VINP_PDKeyAreaLockUnlock_flg/1 -> PMMDataConvert/24(VINP_PDKeyAreaLockUnlock_enum)
  PMMDataConvert/5(VPMM_AllDoorClosed_flg) -> [VPMM_AllDoorClosed_flg]
  PMMDataConvert/10(VPMM_BrkPedalRisingEdge_flg) -> [VPMM_BrkPedalRisingEdge_flg]
  PMMDataConvert/4(VPMM_PreChrgChk_flg) -> [VPMM_PreChrgChk_flg]
  PMM_State_Machine/9(VPMM_HVSysReadyToCharge_enum) -> VPMM_HVSysReadyToCharge_enum/1  "VPMM_HVSysReadyToCharge_enum"
  PMMDataConvert/1(VPMM_DetectDoorOpened_flg) -> [VPMM_DetectDoorOpened_flg]
  PMMDataConvert/2(VPMM_DetectDoorClosed_flg) -> Terminator1/1
  [task_time_s] -> PMMDataConvert/1(task_time_s)
  PMMDataConvert/3(VPMM_BrkPedalPressed_flg) -> [VPMM_BrkPedalPressed_flg]
  PMMDataConvert/9(VPMM_PDKeySta_enum) -> [VPMM_PDKeySta_enum]
  PMM_State_Machine/10(VPMM_PowerSta_enum) -> [VPMM_PowerSta_enum]  "VPMM_PowerSta_enum"
  PMMDataConvert/8(VPMM_MCUReady_flg) -> [VPMM_MCUReady_flg]
  PMMDataConvert/6(VPMM_MCUEnable_flg) -> [VPMM_MCUEnable_flg]
  VINP_PowerOffTSet_cnt/1 -> Gain/1
  Gain/1 -> [VPMM_PowerOffTSet_s]  "VPMM_PowerOffTSet_s"
  VINP_DrivetrainSelect_enum/1 -> PMMDataConvert/36(VINP_DrivetrainSelect_enum)
  PMMDataConvert/21(VPMM_DetectAntitheftUnlock_flg) -> [VPMM_DetectAntitheftUnlock_flg]
  [VPMM_DetectAntitheftUnlock_flg] -> PMM_State_Machine/10(VPMM_DetectAntitheftUnlock_flg)
  PMM_State_Machine/19(VPMM_PreOFF_flg) -> [VPMM_PreOFF_flg]  "VPMM_PreOFF_flg"
  [VPMM_PreOFF_flg] -> Unit Delay10/1
  Unit Delay10/1 -> RequirementManagementForPowerUp/26(VPMM_PreOFF_flg)
  VDHP_ActAPSPosn_pct/1 -> PMM_State_Machine/62(VDHP_ActAPSPosn_pct)
  VINP_FASpeed_kph/1 -> [VINP_FASpeed_kph]
  [VINP_FASpeed_kph] -> RequirementManagementForPowerUp/8(VINP_VehSpeed_kph)
  [VINP_FASpeed_kph] -> PMM_State_Machine/66(VINP_VehSpeed_kph)
  Constant23/1 -> PMM_State_Machine/67(KPMM_APSAllowThd_pct)
  Constant31/1 -> PMM_State_Machine/68(KPMM_PluginVehSpdThd_kph)
  PMMDataConvert/7(VPMM_MCUDischrgFinished_flg) -> Terminator2/1
  VINP_DCDCFaultSta_enum/1 -> PMMDataConvert/37(VINP_DCDCFaultSta_enum)
  [VINP_ChrgPlugSta_enum] -> PMMDataConvert/25(VINP_ChrgPlugSta_enum)
  [VINP_OBCReady4Pre_flg] -> PMMDataConvert/22(VINP_OBCReady4Pre_flg)
  PMMDataConvert/22(VPMM_LVSysErrPwrOutErr_flg) -> VPMM_LVSysErrPwrOutErr_flg/1
  PMM_State_Machine/13(VPMM_PwrStaSW_enum) -> [VPMM_SysPowerMode_enum]  "VPMM_SysPowerMode_enum"
  [VPMM_SysPowerMode_enum] -> VPMM_SysPowerMode_enum/1
  [VPMM_PowerSta_enum] -> VPMM_PowerSta_enum/1
  [VPMM_PowerUpState_enum] -> VPMM_PowerUpState_enum/1
  [VPMM_SysPowerMode_enum] -> MCU_EnaReq_Control/1(VPMM_SysPowerMode_enum)
  Ground8/1 -> Data Type Conversion16/1
  VINP_RrEDURealTMTq_Nm/1 -> MCU_EnaReq_Control/4(VINP_RrEDURealTMTq_Nm)
  [VTQD_GearActualPosn_enum] -> MCU_EnaReq_Control/2(VTQD_GearActualPosn_enum)
  VINP_DCDCAuxCur_A/1 -> PMM_State_Machine/73(VINP_DCDCAuxCur_A)
  Constant33/1 -> PMM_State_Machine/70(KPMM_LVChrgHoldT_s)
  Constant34/1 -> PMM_State_Machine/71(KPMM_SysBaseCurr_A)
  Constant32/1 -> PMM_State_Machine/69(KPMM_LVChrgCurrMthd_flg)
  VINP_FDEWP1Cmd_enum/1 -> PMM_State_Machine/74(VINP_FDEWP1Cmd_enum)
  VINP_FDEWP3Cmd_enum/1 -> PMM_State_Machine/75(VINP_FDEWP3Cmd_enum)
  VINP_CoolgFanActDuty_pct/1 -> PMM_State_Machine/72(VINP_CoolgFanActDuty_pct)
  PMM_State_Machine/20(VPMM_LVSilentChrgSta_enum) -> [VPMM_LVSilentChrgSta_enum]  "VPMM_LVSilentChrgSta_enum"
  [VPMM_LVSilentChrgSta_enum] -> Unit Delay9/1
  Unit Delay9/1 -> RequirementManagementForPowerDown/15(VPMM_LVSilentChrgSta_enum)
  Constant35/1 -> RequirementManagementForPowerDown/16(KPMM_HVSOCWarnTime_s)
  PMMDataConvert/23(VPMM_DetectPDKeyUnlock_flg) -> [VPMM_DetectPDKeyUnlock_flg]
  [VPMM_DetectPDKeyUnlock_flg] -> PMM_State_Machine/76(VPMM_DetectPDKeyUnlock_flg)
  PMMDataConvert/24(VPMM_DetectAntitheftLock_flg) -> [VPMM_DetectAntitheftLock_flg]
  [VPMM_DetectAntitheftLock_flg] -> PMM_State_Machine/77(VPMM_DetectAntitheftLock_flg)
  PMMDataConvert/25(VPMM_DetectPDKeyLock_flg) -> [VPMM_DetectPDKeyLock_flg]
  [VPMM_DetectPDKeyLock_flg] -> PMM_State_Machine/78(VPMM_DetectPDKeyLock_flg)
  VINP_IVIPwroffreq_flg/1 -> [VINP_IVIPwroffreq_flg]
  [VINP_IVIPwroffreq_flg] -> PMM_State_Machine/42(VINP_IVIPwroffreq_flg)
  VINP_SchedChgwake_flg/1 -> [VINP_SchedChgwake_flg]
  [VINP_SchedChgwake_flg] -> RequirementManagementForPowerUp/7(VINP_SchedChgwake_flg)
  [VINP_IVIPwroffreq_flg] -> PMMDataConvert/38(VINP_IVIPwroffreq_flg)
  [VINP_SchedChgwake_flg] -> PMMDataConvert/39(VINP_SchedChgwake_flg)
  PMMDataConvert/26(VPMM_DetectIVIPwroffreq_flg) -> [VPMM_DetectIVIPwroffreq_flg]
  PMMDataConvert/27(VPMM_DetectSchedChg_flg) -> [VPMM_DetectSchedChg_flg]
  VINP_PWCONTINUEUSE_flg/1 -> PMMDataConvert/40(VINP_PWCONTINUEUSE_flg)
  PMMDataConvert/28(VPMM_DetectPWCONTINUE_flg) -> [VPMM_DetectPWCONTINUE_flg]
  [VPMM_DetectPWCONTINUE_flg] -> PMM_State_Machine/81(VPMM_DetectPWCONTINUE_flg)
  [VPMM_DetectIVIPwroffreq_flg] -> PMM_State_Machine/79(VPMM_DetectIVIPwroffreq_flg)
  [VPMM_DetectSchedChg_flg] -> PMM_State_Machine/80(VPMM_DetectSchedChg_flg)
  [VINP_EvccAplusPwrUpReq_flg] -> Data Type Conversion/1
  Data Type Conversion/1 -> VPMM_EvccAplusPwrUpReq_flg/1  "VPMM_EvccAplusPwrUpReq_flg"
  PMM_State_Machine/21(VPMM_PwrStaONTOPopReq_flg) -> VPMM_PwrStaONTOPopReq_flg/1  "VPMM_PwrStaONTOPopReq_flg"
  PMM_State_Machine/22(VPMM_IVIPwrStaONTOPopT_s) -> VPMM_IVIPwrStaONTOPopT_s/1  "VPMM_IVIPwrStaONTOPopT_s"
  PMM_State_Machine/23(VPMM_LVChrgHoldTtimer_s) -> VPMM_LVChrgHoldTtimer_s/1  "VPMM_LVChrgHoldTtimer_s"
  PMM_State_Machine/24(VPMM_LVBattChrgTimeCnt_s) -> VPMM_LVBattChrgTimeCnt_s/1  "VPMM_LVBattChrgTimeCnt_s"
  Constant36/1 -> PMM_State_Machine/82(KPMM_SilentChrgReqTO_s)
  [VINP_HoodSW_flg] -> RequirementManagementForPowerDown/17(VINP_HoodSW_flg)
  Constant37/1 -> PMM_State_Machine/83(KPMM_PwrStaONTOPop_s)
  PMM_State_Machine/26(VPMM_SilentChkAllowSleep_flg) -> VPMM_SilentChkAllowSleep_flg/1  "VPMM_SilentChkAllowSleep_flg"
  PMM_State_Machine/27(VPMM_TimerAllowSleep_flg) -> VPMM_TimerAllowSleep_flg/1  "VPMM_TimerAllowSleep_flg"
  Data Type Conversion39/1 -> VPMM_FDADC12VDetAvg_mV/1  "VPMM_FDADC12VDetAvg_mV"
  PMM_State_Machine/28(VPMM_FDADC12VDetAvg_mV) -> Gain2/1
  PMM_State_Machine/25(VPMM_PMMAllowECUSleep_flg) -> VPMM_PMMAllowECUSleep_flg/1  "VPMM_PMMAllowECUSleep_flg"
  PMM_State_Machine/29(VPMM_LVSilentChrgLv_enum) -> VPMM_LVSilentChrgLv_enum/1  "VPMM_LVSilentChrgLv_enum"
  Constant39/1 -> PMM_State_Machine/88(KPMM_LVBattOFFSlpThd_mV)
  Constant40/1 -> PMM_State_Machine/89(KPMM_OFFLVBattChkRetry_cnt)
  Constant14/1 -> PMM_State_Machine/86(KPMM_FirstLVCheckHoldT_s)
  Constant12/1 -> PMM_State_Machine/85(KPMM_FDADC12VDetAccu_s)
  Constant38/1 -> PMM_State_Machine/87(KPMM_LVBattChkWakehold_s)
  Constant6/1 -> PMM_State_Machine/84(KPMM_FDADC12VDetAccuIntval_s)
  VINP_CANMsgValidBMS5_flg/1 -> PMM_State_Machine/91(VINP_CANMsgValidBMS5_flg)
  Gain2/1 -> Data Type Conversion39/1
  PMM_State_Machine/1(VPMM_PowerUpState_enum) -> [VPMM_PowerUpState_enum]  "VPMM_PowerUpState_enum"
  PMM_State_Machine/2(VPMM_PowerDownState_enum) -> VPMM_PowerDownState_enum/1  "VPMM_PowerDownState_enum"
  PMM_State_Machine/3(VPMM_PowerUpFault_enum) -> VPMM_PowerUpFault_enum/1  "VPMM_PowerUpFault_enum"
  PMM_State_Machine/4(VPMM_PowerDownFault_enum) -> VPMM_PowerDownFault_enum/1  "VPMM_PowerDownFault_enum"
  PMM_State_Machine/5(VPMM_ActiveDischargeReq_flg) -> VPMM_ActiveDischargeReq_flg/1  "VPMM_ActiveDischargeReq_flg"
  [VPMM_SysPowerMode_enum] -> Unit Delay13/1
  [VINP_RePwrReqTbox_enum] -> RequirementManagementForPowerStateConstrain/10(VINP_RePwrReqTbox_enum)
  [VINP_RePwrReqDKCT_enum] -> RequirementManagementForPowerStateConstrain/9(VINP_RePwrReqDKCT_enum)
  [VINP_PwrReq_OTA_enum] -> RequirementManagementForPowerStateConstrain/8(VINP_PwrReq_OTA_enum)
  [VINP_PowerOffTSetDKC_enum] -> RequirementManagementForPowerStateConstrain/7(VPMM_PowerOffTSetDKC_enum)
  [VPMM_PowerOffTSet_s] -> RequirementManagementForPowerStateConstrain/6(VPMM_PowerOffTSet_s)
  [VINP_HVBPreheatPrecoolSta_enum] -> RequirementManagementForPowerStateConstrain/4(VINP_HVBPreheatPrecoolSta_enum)
  VINP_AVMOFFRecButt_flg/1 -> RequirementManagementForPowerStateConstrain/3(VINP_AVMOFFRecButt_flg)
  Unit Delay11/1 -> RequirementManagementForPowerDown/6(VPMM_PwrStaConstraint_enum)
  Unit Delay12/1 -> RequirementManagementForPowerDown/9(VPMM_TCountSta_enum)
  Unit Delay13/1 -> RequirementManagementForPowerStateConstrain/11(VPMM_PwrStaSW_enum)
  [VPMM_LVSilentChrgSta_enum] -> VPMM_LVSilentChrgSta_enum/1
  [VPMM_LVSilentChrgReq_flg] -> VPMM_LVSilentChrgReq_flg/1
  [VINP_TailgateSW_flg] -> PMM_State_Machine/97(VINP_TailgateSW_flg)
  VINP_BMSWarn6_flg/1 -> [VINP_BMSWarn6_flg]
  [VINP_BMSWarn6_flg] -> PMMDataConvert/33(VINP_BMSWarn6_flg)
  [VINP_BMSWarn6_flg] -> PMM_State_Machine/96(VINP_BMSWarn6_flg)
  [VPMM_HVPwrSta_flg] -> VPMM_HVPwrSta_flg/1
  [VPMM_AllDoorClosed_flg] -> RequirementManagementForPowerDown/18(VPMM_AllDoorClosed_flg)
  [VINP_SeatSW_flg] -> RequirementManagementForPowerDown/20(VINP_SeatSW_flg)
  [VPMM_HVPwrSta_flg] -> Unit Delay14/1
  PMMDataConvert/29(VPMM_DetectHVPwrSta_flg) -> [VPMM_DetectHVPwrSta_flg]
  [VPMM_DetectHVPwrSta_flg] -> RequirementManagementForPowerDown/19(VPMM_DetectHVPwrSta_flg)
  Constant41/1 -> RequirementManagementForPowerDown/21(KPMM_SysPwrDownDbns_s)
  Constant43/1 -> PMM_State_Machine/93(KPMM_BattUpResetSW_flg)
  Constant44/1 -> PMM_State_Machine/94(KPMM_BattUpResetTO_s)
  Constant45/1 -> PMM_State_Machine/95(KPMM_BattUpRstDlyTO_s)
  Constant42/1 -> PMM_State_Machine/92(KPMM_BattUpResetRty_cnt)
  PMM_State_Machine/32(VPMM_CtrlFrEDUINVERTER_flg) -> VPMM_CtrlFrEDUINVERTER_flg/1  "VPMM_CtrlFrEDUINVERTER_flg"
  PMM_State_Machine/33(VPMM_CtrlFrPwrStbA1P_flg) -> VPMM_CtrlFrPwrStbA1P_flg/1  "VPMM_CtrlFrPwrStbA1P_flg"
  PMM_State_Machine/34(VPMM_CtrlFrRC1_flg) -> VPMM_CtrlFrRC1_flg/1  "VPMM_CtrlFrRC1_flg"
  PMM_State_Machine/35(VPMM_HWResetSta_enum) -> VPMM_HWResetSta_enum/1  "VPMM_HWResetSta_enum"
  PMM_State_Machine/36(VPMM_HVChrgPreActionErrSta_enum) -> VPMM_HVChrgPreActionErrSta_enum/1  "VPMM_HVChrgPreActionErrSta_enum"
  PMM_State_Machine/30(VPMM_CtrlDrPwrStbA2_flg) -> VPMM_CtrlDrPwrStbA2_flg/1  "VPMM_CtrlDrPwrStbA2_flg"
  PMM_State_Machine/31(VPMM_CtrlFrBMSCCUCIR_flg) -> VPMM_CtrlFrBMSCCUCIR_flg/1  "VPMM_CtrlFrBMSCCUCIR_flg"
  PMMDataConvert/30(VPMM_MCUReady4Pre_flg) -> VPMM_MCUReady4Pre_flg/1
  [VPMM_SafetyChkMLv_flg] -> VPMM_SafetyChkMLv_flg/1
  [VPMM_SafetyChkHLv_flg] -> VPMM_SafetyChkHLv_flg/1
  [VPMM_MCUReady_flg] -> VPMM_MCUReady_flg/1
  Unit Delay14/1 -> PMMDataConvert/41(VPMM_HVPwrSta_flg)
  [VPMM_BrkPedalPressed_flg] -> RequirementManagementForPowerDown/22(VPMM_BrkPedalPressed_flg)
  [VPMM_PwrStaTOSta_enum] -> VPMM_PwrStaTOSta_enum/1
  Constant46/1 -> PMM_State_Machine/98(KPMM_HoodOffChkFailtime_s)
  Constant28/1 -> RequirementManagementForPowerDown/24(KPMM_HVBattSOCPwrDwnThd_pct)
  [VINP_EvccAplusPwrUpReq_flg] -> RequirementManagementForPowerDown/23(VINP_EvccAplusPwrUpReq_flg)
  [VPMM_PowerSta_enum] -> DCDC output volt setpoint judgment/2(VPMM_PowerSta_enum)
  [VPMM_HVPwrSta_flg] -> DCDC output volt setpoint judgment/3(VPMM_HVPwrSta_flg)
  [VPMM_LVSilentChrgReq_flg] -> DCDC output volt setpoint judgment/4(VPMM_LVSilentChrgReq_flg)
  [VPMM_LVSilentChrgReqStd_flg] -> DCDC output volt setpoint judgment/5(VPMM_LVSilentChrgReqStd_flg)
  DCDC output volt setpoint judgment/1(VPMM_DCDCVoltSetpoint_V) -> VPMM_DCDCVoltSetpoint_V/1  "VPMM_DCDCVoltSetpoint_V"
  PMM_State_Machine/7(VPMM_DCDCVoltSetpointPU_V) -> [VPMM_DCDCVoltSetpointPU_V]  "VPMM_DCDCVoltSetpointPU_V"
  [VPMM_DCDCVoltSetpointPU_V] -> DCDC output volt setpoint judgment/1(VPMM_DCDCVoltSetpointPU_V)
  Constant27/1 -> PMM_State_Machine/99(KPMM_HVSOCWarnThd_pct)
  VINP_OFFACMODE_enum/1 -> [VINP_OFFACMODE_enum]
  [VINP_OFFACMODE_enum] -> RequirementManagementForPowerStateConstrain/5(VINP_OFFACMODE_enum)
  [VINP_OFFACMODE_enum] -> PMM_State_Machine/100(VINP_OFFACMODE_enum)
  VINP_V2LSta_enum/1 -> PMM_State_Machine/101(VINP_V2LSta_enum)
  Ground10/1 -> Cast To Boolean/1
  Ground11/1 -> Cast To Boolean1/1
  Ground12/1 -> Cast To Boolean2/1
  [VINP_PsDoorSW_flg] -> PMMDataConvert/4(VINP_PsDoorSW_flg)
  [VINP_RRDoorSW_flg] -> PMMDataConvert/5(VINP_RRDoorSW_flg)
  [VINP_RLDoorSW_flg] -> PMMDataConvert/6(VINP_RLDoorSW_flg)
  [VINP_PsDoorSW_flg] -> PMM_State_Machine/102(VINP_PsDoorSW_flg)
  [VINP_RRDoorSW_flg] -> PMM_State_Machine/103(VINP_RRDoorSW_flg)
  [VINP_RLDoorSW_flg] -> PMM_State_Machine/104(VINP_RLDoorSW_flg)
  [VINP_RLDoorSW_flg] -> Detect Increase2/1
  [VINP_RRDoorSW_flg] -> Detect Increase1/1
  [VINP_PsDoorSW_flg] -> Detect Increase/1
  [VINP_SeatSW_flg] -> Detect Decrease/1
  Detect Decrease/1 -> PMM_State_Machine/108(VPMM_DetectSeatEmpty_flg)  "VPMM_DetectSeatEmpty_flg"
  Detect Increase/1 -> PMM_State_Machine/105(VPMM_DetectPsDoorOpened_flg)  "VPMM_DetectPsDoorOpened_flg"
  Detect Increase2/1 -> PMM_State_Machine/106(VPMM_DetectRLDoorOpened_flg)  "VPMM_DetectRLDoorOpened_flg"
  Detect Increase1/1 -> PMM_State_Machine/107(VPMM_DetectRRDoorOpened_flg)  "VPMM_DetectRRDoorOpened_flg"
  VINP_LVBattDet12V_V/1 -> Data Type Conversion1/1
  Data Type Conversion1/1 -> PMM_State_Machine/24(VINP_LVBattDet12V_V), [VINP_LVBattDet12V_V]
  PMM_State_Machine/37(VPMM_PMMAllowNMSleep_flg) -> VPMM_PMMAllowNMSleep_flg/1  "VPMM_PMMAllowNMSleep_flg"
  Gain1/1 -> Data Type Conversion2/1
  [VINP_LVBattDet12V_V] -> Gain1/1
  Data Type Conversion2/1 -> PMM_State_Machine/90(VINP_LvBattVolt_mV)
  VDKC_KeyAreaLockUnlock_enum/1 -> PMMDataConvert/42(VDKC_KeyAreaLockUnlock_enum)
  VDKC_KeyAreaPS_enum/1 -> PMMDataConvert/43(VDKC_KeyAreaPS_enum)
  VINP_CANMsgValidDKC1_flg/1 -> PMMDataConvert/44(VINP_CANMsgValidDKC1_flg)
  VINP_PDKeyAreaPS_flg/1 -> PMMDataConvert/45(VINP_PDKeyAreaPS_enum)
  [VPMM_PowerSta_enum] -> Unit Delay15/1
  Unit Delay15/1 -> Data Type Conversion3/1
  Data Type Conversion3/1 -> PushButton_Handle/1(VPMM_PowerStaLast_enum)
  [VINP_PBSWGPIO_flg] -> PushButton_Handle/2(VINP_PBSWGPIO_flg)
  PMM_State_Machine/38(VPMM_DCDCRlyDem_enum) -> VPMM_DCDCRlyDem_enum/1  "VPMM_DCDCRlyDem_enum"
  PMM_State_Machine/39(VPMM_EACRlyDem_enum) -> VPMM_EACRlyDem_enum/1  "VPMM_EACRlyDem_enum"
  PMM_State_Machine/40(VPMM_DCDCEnDem_enum) -> VPMM_DCDCEnDem_enum/1  "VPMM_DCDCEnDem_enum"
  PMM_State_Machine/41(VPMM_EHPSRlyDem_enum) -> VPMM_EHPSRlyDem_enum/1  "VPMM_EHPSRlyDem_enum"
  PushButton_Handle/1(VPMM_OFFPBPRess_flg) -> [VPMM_OFFPBPress_flg]
  PushButton_Handle/2(VPMM_STBPBPRess_flg) -> [VPMM_STBPBPress_flg]
  PushButton_Handle/3(VPMM_ONPBPRess_flg) -> [VPMM_ONPBPress_flg]
  PushButton_Handle/4(VPMM_READYPBPRess_flg) -> [VPMM_READYPBPress_flg]
  PushButton_Handle/5(VPMM_OFFAPBPRess_flg) -> [VPMM_OFFAPBPress_flg]
  PushButton_Handle/6(VPMM_OFFCPBPRess_flg) -> [VPMM_OFFCPBPress_flg]
  [VPMM_OFFPBPress_flg] -> PMM_State_Machine/115(VPMM_OFFPBRisingEdge_flg)
  [VPMM_STBPBPress_flg] -> PMM_State_Machine/116(VPMM_STBPBRisingEdge_flg)
  [VPMM_ONPBPress_flg] -> PMM_State_Machine/117(VPMM_ONPBRisingEdge_flg)
  [VPMM_READYPBPress_flg] -> PMM_State_Machine/119(VPMM_READYPBRisingEdge_flg)
  [VPMM_OFFAPBPress_flg] -> PMM_State_Machine/120(VPMM_OFFAPBRisingEdge_flg)
  [VPMM_OFFCPBPress_flg] -> PMM_State_Machine/121(VPMM_OFFCPBRisingEdge_flg)
  [VPMM_OFFPBPress_flg] -> RequirementManagementForPowerUp/27(VPMM_OFFPBPress_flg)
  PushButton_Handle/7(VPMM_ONPBSta_flg) -> [VPMM_ONPBSta_flg]
  [VPMM_ONPBSta_flg] -> PMM_State_Machine/118(VPMM_ONPBSta_flg)
  [VPMM_STBPBPress_flg] -> RequirementManagementForPowerUp/28(VPMM_STBPBPress_flg)
  Constant47/1 -> PMM_State_Machine/125(KPMM_FDADC24VDetAccu_s)
  Constant48/1 -> PMM_State_Machine/124(KPMM_FDADC24VDetAccuIntval_s)
  Constant49/1 -> PMM_State_Machine/123(KPMM_LVBattOFFSlpThd24V_mV)
  [VINP_LVBattDet24V_V] -> Gain3/1, PMM_State_Machine/128(VINP_LVBattDet24V_V)
  Gain3/1 -> Data Type Conversion4/1
  Data Type Conversion4/1 -> PMM_State_Machine/122(VINP_LvBattVolt24V_mV)
  Constant50/1 -> PMM_State_Machine/127(KPMM_LVBattThd24V_V)
  [VINP_CANMsgValidDCDCStatus2_flg] -> PMM_State_Machine/126(VINP_CANMsgValidDCDCStatus2_flg)
  [VINP_PDUDCDCRlySta_enum] -> PMM_State_Machine/109(VINP_PDUDCDCRlySta_enum)
  [VINP_PDUEACRlySta_enum] -> PMM_State_Machine/110(VINP_PDUEACRlySta_enum)
  [VINP_DCDCEnSta_enum] -> PMM_State_Machine/111(VINP_DCDCEnSta_enum)
  [VINP_PDUEHPSRlySta_enum] -> PMM_State_Machine/112(VINP_PDUEHPSRlySta_enum)
  [VINP_EACEnSta_enum] -> PMM_State_Machine/113(VINP_EACEnSta_enum)
  [VINP_EHPSEnSta_enum] -> PMM_State_Machine/114(VINP_EHPSEnSta_enum)
  VINP_PBSWGPIO_flg/1 -> [VINP_PBSWGPIO_flg]
  VINP_PDUDCDCRlySta_enum/1 -> [VINP_PDUDCDCRlySta_enum]
  VINP_PDUEACRlySta_enum/1 -> [VINP_PDUEACRlySta_enum]
  VINP_DCDCEnSta_enum/1 -> [VINP_DCDCEnSta_enum]
  VINP_PDUEHPSRlySta_enum/1 -> [VINP_PDUEHPSRlySta_enum]
  VINP_EACEnSta_enum/1 -> [VINP_EACEnSta_enum]
  VINP_EHPSEnSta_enum/1 -> [VINP_EHPSEnSta_enum]
  VINP_CANMsgValidDCDCStatus2_flg/1 -> [VINP_CANMsgValidDCDCStatus2_flg]
  VINP_LVBattDet24V_V/1 -> [VINP_LVBattDet24V_V]
  VINP_PDUSelfChkSta_flg/1 -> [VINP_PDUSelfChkSta_flg]
  [VINP_PDUSelfChkSta_flg] -> PMMDataConvert/46(VINP_PDUSelfChkSta_flg)
  Data Type Conversion5/1 -> BoringSpec/1(VPMM_PowerStaLast_enum)
  Unit Delay16/1 -> Data Type Conversion5/1
  [VPMM_PowerSta_enum] -> Unit Delay16/1
  [VPMM_PDKeySta_enum] -> BoringSpec/2(VPMM_PDKeySta_enum)
  [VINP_SeatSW_flg] -> BoringSpec/3(VINP_SeatSW_flg)
  [VTQD_GearActualPosn_enum] -> BoringSpec/4(VTQD_GearActualPosn_enum)
  [task_time_s] -> BoringSpec/5(task_time_s)
  BoringSpec/1(VPMM_UserLeaveTChk_flg) -> [VPMM_UserLeaveTChk_flg]
  [VPMM_UserLeaveTChk_flg] -> PMM_State_Machine/131(VPMM_UserLeaveTChk_flg)
  [VPMM_READYPBMemory_flg] -> PMM_State_Machine/130(VPMM_READYPBMemory_flg)
  PushButton_Handle/8(VPMM_READYPBMemory_flg) -> [VPMM_READYPBMemory_flg]
  [VINP_FDDoorOpen_enum] -> PMM_State_Machine/132(VINP_FDDoorOpen_enum)
  VINP_FDDoorOpen_enum/1 -> [VINP_FDDoorOpen_enum]
  VINP_EBSBrakeSW_enum/1 -> PMMDataConvert/47(VINP_EBSBrakeSW_enum)
  [VACC_EACPreSelfChkSta_flg] -> PMM_State_Machine/133(VACC_EACPreSelfChkSta_flg)
  VACC_EACPreSelfChkSta_flg/1 -> [VACC_EACPreSelfChkSta_flg]
  Data Type Conversion6/1 -> [VINP_FrTMSpd_rpm]
  Data Type Conversion7/1 -> [VINP_DrDoorSW_flg]
  Data Type Conversion8/1 -> PMMDataConvert/8(VINP_FrMCUDischrgSta_flg)
  Data Type Conversion9/1 -> PMMDataConvert/9(VINP_FrMCUEnaSta_flg)
  Data Type Conversion10/1 -> PMMDataConvert/10(VINP_FrMCUErr_enum)
  Data Type Conversion11/1 -> PMMDataConvert/11(VINP_FrMCUReady4Pre_flg)
  Data Type Conversion12/1 -> PMMDataConvert/12(VINP_FrMCUReady_flg)
  Data Type Conversion13/1 -> PMMDataConvert/13(VINP_FrMCUTemp_C)
  Data Type Conversion14/1 -> PMMDataConvert/7(VINP_FrMCUDCBusVolt_V)
  Data Type Conversion15/1 -> PMMDataConvert/28(VINP_CrashOutputSts_enum)
  Cast To Boolean/1 -> [VINP_PsDoorSW_flg]
  Cast To Boolean1/1 -> [VINP_RRDoorSW_flg]
  Cast To Boolean2/1 -> [VINP_RLDoorSW_flg]
  Data Type Conversion16/1 -> MCU_EnaReq_Control/3(VINP_FrEDURealTMTq_Nm)
  [VINP_FDDoorOpen_enum] -> PMM_State_Machine/129(VINP_FDDoorstate_enum)
  PushButton_Handle/9(VPMM_PwrUpPBPress_flg) -> [VPMM_PwrUpPBPress_flg]
  [VPMM_PwrUpPBPress_flg] -> PMM_State_Machine/134(VPMM_PwrUpPBPress_flg)

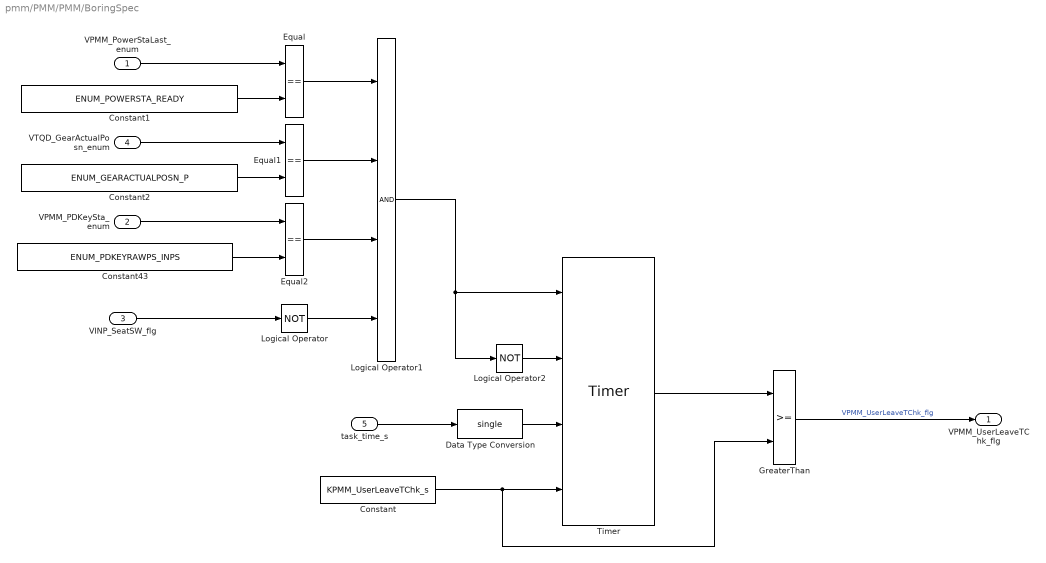
== system pmm/PMM/PMM/BoringSpec ==
  VPMM_PowerStaLast_enum : Inport
  VPMM_PDKeySta_enum : Inport  Port=2
  VINP_SeatSW_flg : Inport  Port=3
  VTQD_GearActualPosn_enum : Inport  Port=4
  task_time_s : Inport  Port=5
  Constant : Constant  Value=KPMM_UserLeaveTChk_s
  Constant1 : Constant  Value=ENUM_POWERSTA_READY
  Constant2 : Constant  Value=ENUM_GEARACTUALPOSN_P
  Constant43 : Constant  Value=ENUM_PDKEYRAWPS_INPS
  Data Type Conversion : DataTypeConversion  OutDataTypeStr=single
  Equal : RelationalOperator  Operator===  OutDataTypeStr=boolean  RndMeth=Simplest
  Equal1 : RelationalOperator  Operator===  OutDataTypeStr=boolean  RndMeth=Simplest
  Equal2 : RelationalOperator  Operator===  OutDataTypeStr=boolean  RndMeth=Simplest
  GreaterThan : RelationalOperator  OutDataTypeStr=boolean  RndMeth=Simplest
  Logical Operator : Logic  Operator=NOT  AllPortsSameDT=off  OutDataTypeStr=boolean
  Logical Operator1 : Logic  Inputs=4  AllPortsSameDT=off  OutDataTypeStr=boolean
  Logical Operator2 : Logic  Operator=NOT  AllPortsSameDT=off  OutDataTypeStr=boolean
  Timer : hcu_lib/Basic_Blocks/Timer
  VPMM_UserLeaveTChk_flg : Outport
  wires:
  task_time_s/1 -> Data Type Conversion/1
  Constant/1 -> GreaterThan/2, Timer/4
  Constant1/1 -> Equal/2
  VPMM_PowerStaLast_enum/1 -> Equal/1
  VTQD_GearActualPosn_enum/1 -> Equal1/1
  Constant2/1 -> Equal1/2
  VPMM_PDKeySta_enum/1 -> Equal2/1
  VINP_SeatSW_flg/1 -> Logical Operator/1
  Constant43/1 -> Equal2/2
  Equal/1 -> Logical Operator1/1
  Equal1/1 -> Logical Operator1/2
  Equal2/1 -> Logical Operator1/3
  Logical Operator/1 -> Logical Operator1/4
  Logical Operator1/1 -> Logical Operator2/1, Timer/1
  Logical Operator2/1 -> Timer/2
  Timer/1 -> GreaterThan/1
  GreaterThan/1 -> VPMM_UserLeaveTChk_flg/1  "VPMM_UserLeaveTChk_flg"
  Data Type Conversion/1 -> Timer/3
